simulink model "current_measure"  (R2024b)
settings: Solver=ode1be  StartTime=0.0  StopTime=simlength  FixedStep=ts  RelTol=1e-3
values from neighbouring files (symbols this model uses):
  ts = 1e-6    (= 1e-06)    [init.m]
libraries: fl_lib x19, nesl_utility x9, ee_lib x2
settings Model: Creator=ltnbda  LastModifiedBy=ltnbda
settings DataIOCC: SaveOutput=off  SignalLogging=off  DSMLogging=off  SaveTime=off  ReturnWorkspaceOutputs=off
settings RTWCC: GPUComputeCapability=3.5

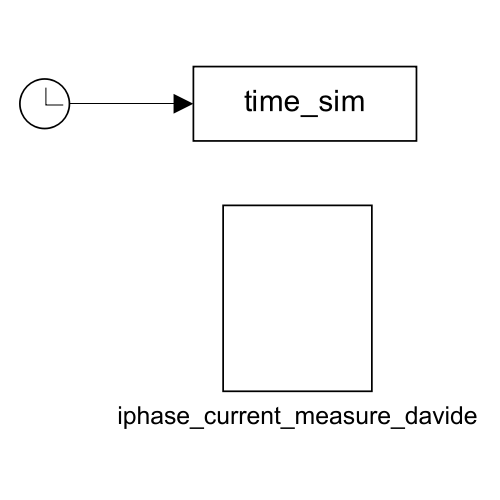
[thumbnail: Simulink's stored preview of the top-level diagram]
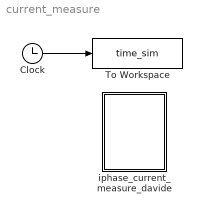
== system current_measure ==
  Clock : Clock
  To Workspace : ToWorkspace  VariableName=time_sim  SampleTime=ts
      settings: MaxDataPoints=N  Save2DSignal=2-D array (concatenate along first dimension)
  iphase_current_measure_davide : Subsystem
  wires:
  Clock/1 -> To Workspace/1

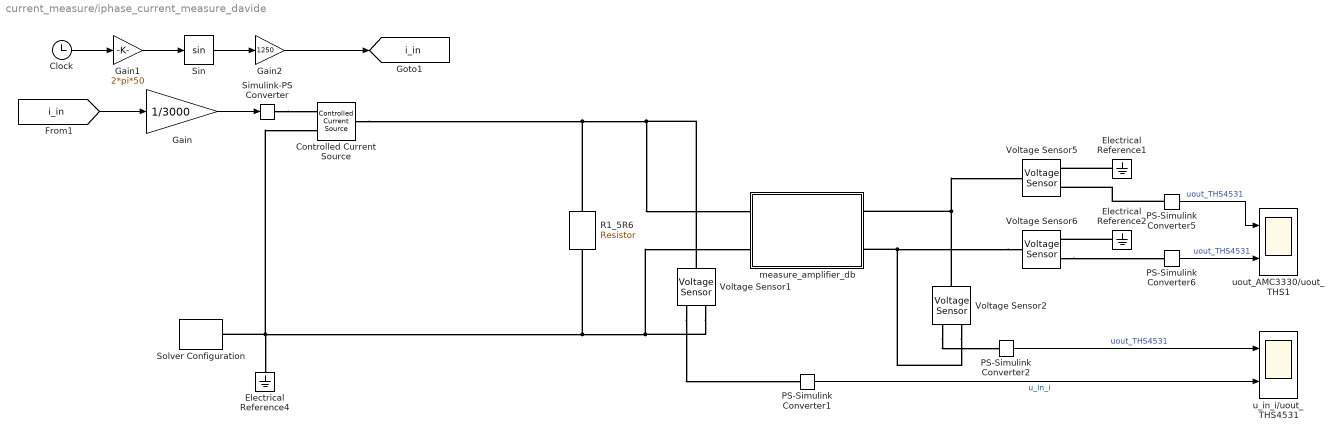
== system current_measure/iphase_current_measure_davide ==
  Clock : Clock
  Controlled Current Source : fl_lib/Electrical/Electrical Sources/Controlled Current Source
  Electrical Reference1 : fl_lib/Electrical/Electrical Elements/Electrical Reference
  Electrical Reference2 : fl_lib/Electrical/Electrical Elements/Electrical Reference
  Electrical Reference4 : fl_lib/Electrical/Electrical Elements/Electrical Reference
  Gain : Gain  Gain=1/3000
  Gain1 : Gain  Gain=2*pi*50
  Gain2 : Gain  Gain=1250
  PS-Simulink Converter{1..2,5..6} (4 alike) : nesl_utility/PS-Simulink Converter  PhysicalDomain=network_engine_domain  SubClassName=ps_output  LeftPortType=input  RightPortType=output  PseudoPeriodic=off  Frequencies=[]  VectorFormat=1-D array  Unit=V  AffineConversion=off
  R1_5R6 : fl_lib/Electrical/Electrical Elements/Resistor  R=5.6 Ohm  i_specify=off  i_priority=None  i=0 A  i_nominal_specify=off  i_nominal_value=1  i_nominal_unit=A  v_specify=off  v_priority=None  v=0 V  v_nominal_specify=off  v_nominal_value=1  v_nominal_unit=V
  Simulink-PS Converter : nesl_utility/Simulink-PS Converter  PhysicalDomain=network_engine_domain  SubClassName=ps_input  LeftPortType=input  RightPortType=output  PseudoPeriodic=off  Frequencies=[]  NoiseDistribution=none  NoiseParameters=[]  Unit=A  AffineConversion=off  FilteringAndDerivatives=provide  SimscapeFilterOrder=1  InputFilterTimeConstant=0.001  UdotUserProvided=0
  Sin : Trigonometry
  Solver Configuration : nesl_utility/Solver Configuration  PhysicalDomain=network_engine_domain  SubClassName=solver  LeftPortType=input  RightPortType=generic  Tones=[]  Harmonics=[]  SimulateNoise=off  Profile=off  UseLocalSampling=off  EnableSwitchedLinearOptims=on  FrequencyDomain=off  UseCCode=off  RelTol=0.001  AbsTol=0.001  MinStep=1e-09  ToWorkspace=off  RevertToSquareIcSolve=off  NumHomotopyIterations=100  PhasorMode=off  PhasorModeNumHarmonics=1  ConsistencySolver=NEWTON_XTOL_AFTER_FTOL  IndexReductionMethod=DerivativeReplacement  DoDC=on  ResidualTolerance=1e-09  ConsistencyTolSource=GLOBAL  ConsistencyAbsTol=0.001  ConsistencyRelTol=0.001  ConsistencyTolFactor=0.001  UseLocalSolver=on  LocalSolverChoice=NE_BACKWARD_EULER_ADVANCER  ResolveIndetEquations=on  FunctionEvalNumThread=1  LocalSolverSampleTime=ts  DoFixedCost=on  MaxNonlinIter=3  MaxModeIter=2  ComputeImpulses=off  ImpulseIterations=2  LinearAlgebra=auto  LinearAlgebraNumThread=0  EquationFormulation=NE_TIME_EF  DelaysMemoryBudget=1024  AutomaticFiltering=on  FilteringTimeConstant=0.001  PartitionStorageMethod=AS_NEEDED  PartitionMemoryBudget=1024  PartitionMethod=ROBUST  MultibodyUseLocalSolver=off  MultibodyLocalSolverChoice=ODE1  MultibodyLocalSolverSampleTime=0.001
  Voltage Sensor{1..2,5..6} (4 alike) : fl_lib/Electrical/Electrical Sensors/Voltage Sensor
  measure_amplifier_db : Subsystem
  u_in_i/uout_THS4531 : Scope  NumInputPorts=2
  uout_AMC3330/uout_THS1 : Scope  NumInputPorts=2
  tag scope: i_in=global
  wires:
  PS-Simulink Converter6/1 -> uout_AMC3330/uout_THS1/2  "uout_THS4531"
  PS-Simulink Converter5/1 -> uout_AMC3330/uout_THS1/1  "uout_THS4531"
  PS-Simulink Converter1/1 -> u_in_i/uout_THS4531/2  "u_in_i"
  Gain/1 -> Simulink-PS Converter/1
  PS-Simulink Converter2/1 -> u_in_i/uout_THS4531/1  "uout_THS4531"
  [i_in] -> Gain/1
  Sin/1 -> Gain2/1
  Gain2/1 -> [i_in]
  Gain1/1 -> Sin/1
  Clock/1 -> Gain1/1
  connections:
  Voltage Sensor6/RConn1 -- PS-Simulink Converter6/LConn1
  PS-Simulink Converter5/LConn1 -- Voltage Sensor5/RConn1
  Electrical Reference2/LConn1 -- Voltage Sensor6/RConn2
  Electrical Reference1/LConn1 -- Voltage Sensor5/RConn2
  Voltage Sensor1/RConn1 -- PS-Simulink Converter1/LConn1
  Voltage Sensor6/LConn1 -- measure_amplifier_db/RConn2 -- Voltage Sensor2/RConn2
  Voltage Sensor1/RConn2 -- measure_amplifier_db/LConn2 -- Electrical Reference4/LConn1 -- Solver Configuration/RConn1 -- Controlled Current Source/RConn2 -- R1_5R6/RConn1
  Voltage Sensor2/RConn1 -- PS-Simulink Converter2/LConn1
  measure_amplifier_db/RConn1 -- Voltage Sensor5/LConn1 -- Voltage Sensor2/LConn1
  Simulink-PS Converter/RConn1 -- Controlled Current Source/RConn1
  Voltage Sensor1/LConn1 -- Controlled Current Source/LConn1 -- R1_5R6/LConn1 -- measure_amplifier_db/LConn1

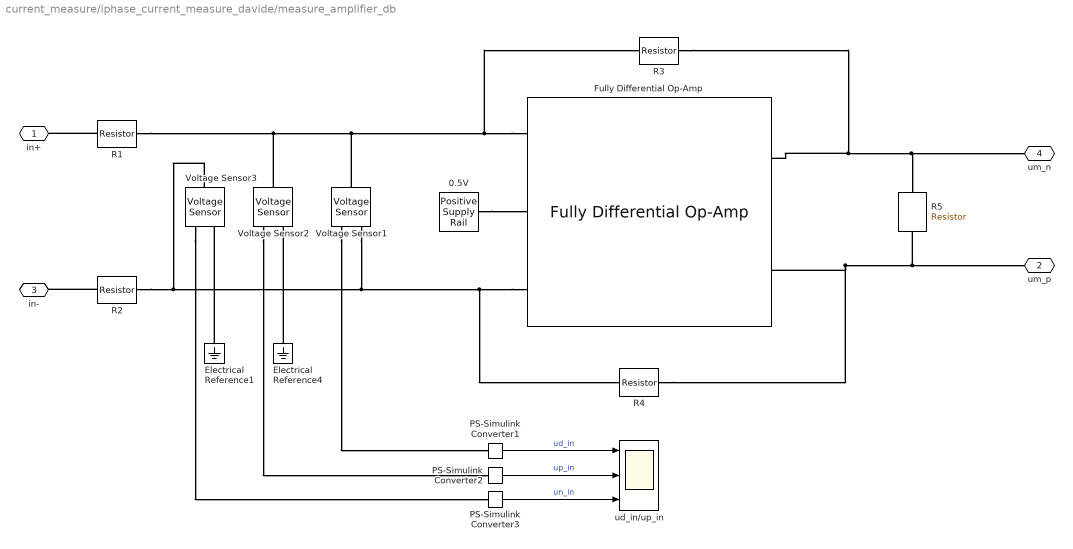
== system current_measure/iphase_current_measure_davide/measure_amplifier_db ==
  0.5V : ee_lib/Sources/Positive Supply Rail  v0=0.5 V
      settings: InternalSimscapePortConfiguration="{\"Bottom\":[],\"Left\":[],\"Right\":[{\"id\":\"p\",\"label\":\"\",\"type\":\"foundation.electrical.electrical\"}],\"Top\":[]}"
  Electrical Reference1 : fl_lib/Electrical/Electrical Elements/Electrical Reference
  Electrical Reference4 : fl_lib/Electrical/Electrical Elements/Electrical Reference
  Fully Differential Op-Amp : ee_lib/Integrated Circuits/Fully Differential Op-Amp  A=1e3  f=1.5 GHz  Rdiff=1.3 MOhm  Cdiff=1.8 pF  Rcom=1.0 MOhm  Ccom=2.3 pF  Rout=1 Ohm  Vmin=-1.4 V  Vmax=1.4 V  Vdotdiff=5000 V/us  Rocm=23.0 kOhm  Vs_neg=-5 V  Vs_pos=5 V  V0=0 V
      settings: InternalSimscapePortConfiguration="{\"Bottom\":[],\"Left\":[{\"id\":\"n\",\"label\":\"-\",\"type\":\"foundation.electrical.electrical\"},{\"id\":\"cm\",\"label\":\"cm\",\"type\":\"foundation.electrical.electrical\"},{\"id\":\"p\",\"label\":\"+\",\"type\":\"foundation.electrical.electrical\"}],\"Right\":[{\"id\":\"out_p\",\"label\":\"+\",\"type\":\"foundation.electrical.electrical\"},{\"id\":\"out_n\",\"label\":\"-\",\"type\":\"foundation.electrical.electrical\"}],\"Top\":[]}"
  PS-Simulink Converter1 : nesl_utility/PS-Simulink Converter  PhysicalDomain=network_engine_domain  SubClassName=ps_output  LeftPortType=input  RightPortType=output  PseudoPeriodic=off  Frequencies=[]  VectorFormat=1-D array  Unit=V  AffineConversion=off
  PS-Simulink Converter2 : nesl_utility/PS-Simulink Converter  PhysicalDomain=network_engine_domain  SubClassName=ps_output  LeftPortType=input  RightPortType=output  PseudoPeriodic=off  Frequencies=[]  VectorFormat=1-D array  Unit=V  AffineConversion=off
  PS-Simulink Converter3 : nesl_utility/PS-Simulink Converter  PhysicalDomain=network_engine_domain  SubClassName=ps_output  LeftPortType=input  RightPortType=output  PseudoPeriodic=off  Frequencies=[]  VectorFormat=1-D array  Unit=V  AffineConversion=off
  R1 : fl_lib/Electrical/Electrical Elements/Resistor  R=4700 Ohm  i_specify=off  i_priority=None  i=0 A  i_nominal_specify=off  i_nominal_value=1  i_nominal_unit=A  v_specify=off  v_priority=None  v=0 V  v_nominal_specify=off  v_nominal_value=1  v_nominal_unit=V
  R2 : fl_lib/Electrical/Electrical Elements/Resistor  R=4700 Ohm  i_specify=off  i_priority=None  i=0 A  i_nominal_specify=off  i_nominal_value=1  i_nominal_unit=A  v_specify=off  v_priority=None  v=0 V  v_nominal_specify=off  v_nominal_value=1  v_nominal_unit=V
  R3 : fl_lib/Electrical/Electrical Elements/Resistor  R=1e3 %940 Ohm  i_specify=off  i_priority=None  i=0 A  i_nominal_specify=off  i_nominal_value=1  i_nominal_unit=A  v_specify=off  v_priority=None  v=0 V  v_nominal_specify=off  v_nominal_value=1  v_nominal_unit=V
  R4 : fl_lib/Electrical/Electrical Elements/Resistor  R=1e3 %940 Ohm  i_specify=off  i_priority=None  i=0 A  i_nominal_specify=off  i_nominal_value=1  i_nominal_unit=A  v_specify=off  v_priority=None  v=0 V  v_nominal_specify=off  v_nominal_value=1  v_nominal_unit=V
  R5 : fl_lib/Electrical/Electrical Elements/Resistor  R=2e3 Ohm  i_specify=off  i_priority=None  i=0 A  i_nominal_specify=off  i_nominal_value=1  i_nominal_unit=A  v_specify=off  v_priority=None  v=0 V  v_nominal_specify=off  v_nominal_value=1  v_nominal_unit=V
  Voltage Sensor1 : fl_lib/Electrical/Electrical Sensors/Voltage Sensor
  Voltage Sensor2 : fl_lib/Electrical/Electrical Sensors/Voltage Sensor
  Voltage Sensor3 : fl_lib/Electrical/Electrical Sensors/Voltage Sensor
  ud_in/up_in : Scope  NumInputPorts=3
  in+ : PMIOPort  Side=Left
  um_p : PMIOPort  Port=2  Side=Right
  in- : PMIOPort  Port=3  Side=Left
  um_n : PMIOPort  Port=4  Side=Right
  wires:
  PS-Simulink Converter3/1 -> ud_in/up_in/3  "un_in"
  PS-Simulink Converter2/1 -> ud_in/up_in/2  "up_in"
  PS-Simulink Converter1/1 -> ud_in/up_in/1  "ud_in"
  connections:
  Voltage Sensor3/RConn1 -- PS-Simulink Converter3/LConn1
  Electrical Reference1/LConn1 -- Voltage Sensor3/RConn2
  Voltage Sensor2/RConn1 -- PS-Simulink Converter2/LConn1
  Electrical Reference4/LConn1 -- Voltage Sensor2/RConn2
  Voltage Sensor1/RConn1 -- PS-Simulink Converter1/LConn1
  R5/RConn1 -- um_p/RConn1 -- Fully Differential Op-Amp/RConn1 -- R4/RConn1
  Fully Differential Op-Amp/RConn2 -- R5/LConn1 -- um_n/RConn1 -- R3/RConn1
  0.5V/RConn1 -- Fully Differential Op-Amp/LConn2
  Fully Differential Op-Amp/LConn1 -- R4/LConn1 -- Voltage Sensor1/RConn2 -- Voltage Sensor3/LConn1 -- R2/RConn1
  R2/LConn1 -- in-/RConn1
  Fully Differential Op-Amp/LConn3 -- R3/LConn1 -- Voltage Sensor1/LConn1 -- Voltage Sensor2/LConn1 -- R1/RConn1
  R1/LConn1 -- in+/RConn1
